simulink model "atm"  (R2017a)
settings: Solver=FixedStepDiscrete  StartTime=0.0  StopTime=15  FixedStep=0.1  RelTol=1e-3  EnableMultiTasking=on
settings Model: NumberOfSteps=10  Creator=thr  LastModifiedBy=thr
settings SolverCC: AutoInsertRateTranBlk=on
settings DataIOCC: LimitDataPoints=on
settings OptimizationCC: LifeSpan=inf
settings DebuggingCC: AllowSymbolicDim=off  SFUnexpectedBacktrackingDiag=warning  SFNoUnconditionalDefaultTransitionDiag=warning  SFExecutionAtInitializationDiag=none
settings GRTTargetCC: TargetLangStandard=C89/C90 (ANSI)  GeneratePreprocessorConditionals=Disable all
settings ConfigComp: CovMetricSettings=dw  CovHtmlReporting=on  CovSaveCumulativeToWorkspaceVar=on  CovSaveSingleToWorkspaceVar=on  CovShowResultsExplorer=off  CovExternalEMLEnable=off  CovSFcnEnable=off

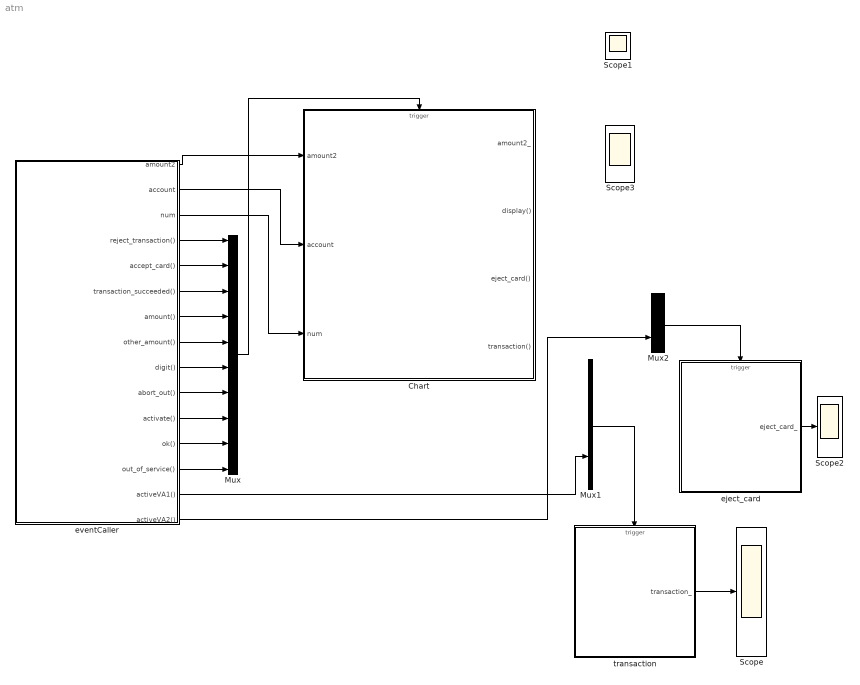
== system atm ==
  Chart : Stateflow chart  TreatAsAtomicUnit=on
  Mux : Mux  Inputs=10
  Mux1 : Mux  Inputs=2
  Mux2 : Mux  Inputs=2
  Scope : Scope
  Scope1 : Scope
  Scope2 : Scope
  Scope3 : Scope  NumInputPorts=2
  eject_card : Stateflow chart  TreatAsAtomicUnit=on
  eventCaller : Stateflow chart  TreatAsAtomicUnit=on
  transaction : Stateflow chart  TreatAsAtomicUnit=on
  wires:
  eventCaller/1(amount2) -> Chart/1(amount2)
  eventCaller/2(account) -> Chart/2(account)
  eventCaller/3(num) -> Chart/3(num)
  Mux/1 -> Chart/Trigger
  eventCaller/4(reject_transaction()) -> Mux/1
  eventCaller/5(accept_card()) -> Mux/2
  eventCaller/6(transaction_succeeded()) -> Mux/3
  eventCaller/7(amount()) -> Mux/4
  eventCaller/8(other_amount()) -> Mux/5
  eventCaller/9(digit()) -> Mux/6
  eventCaller/10(abort_out()) -> Mux/7
  eventCaller/11(activate()) -> Mux/8
  eventCaller/12(ok()) -> Mux/9
  eventCaller/13(out_of_service()) -> Mux/10
  Mux1/1 -> transaction/Trigger
  eventCaller/14(activeVA1()) -> Mux1/2
  transaction/1(transaction_) -> Scope/1
  eventCaller/15(activeVA2()) -> Mux2/2
  Mux2/1 -> eject_card/Trigger
  eject_card/1(eject_card_) -> Scope2/1

== stateflow chart atm/eventCaller ==
  state S1
  state S2
  state S3
  state S5
  state S4
  state S6
  state S10
  state S9
  state S8
  state S14
  state S7
  state S11
  (default) -> S1 : {activate, activeVA1,activeVA2}
  S2 -> S3 : after(1, sec)
      | {amount2=5000,
      | amount}
  S1 -> S2 : after(1, sec)
      | {accept_card,
      | account=2345}
  S3 -> S5 : after(1, sec)
      | {reject_transaction}
  S5 -> S4 : after(1, sec)
      | {num=5,
      | digit}
  S4 -> S6 : after(1, sec)
      | {num=0,
      | digit}
  S6 -> S7 : after(1, sec)
      | {num=0,
      | digit}
  S8 -> S9 : after(1, sec)
      | {num=5,
      | digit}
  S14 -> S8 : after(1, sec)
      | {reject_transaction}
  S7 -> S14 : after(1, sec)
      | {ok}
  S9 -> S10 : after(1, sec)
      | {ok}
  S10 -> S11 : after(1, sec)
      | {transaction_succeeded}
  data: amount2 output int32; account output int32; num output int32
  events: reject_transaction output FUNCTION_CALL_EVENT; accept_card output FUNCTION_CALL_EVENT; transaction_succeeded output FUNCTION_CALL_EVENT; amount output FUNCTION_CALL_EVENT; other_amount output FUNCTION_CALL_EVENT; digit output FUNCTION_CALL_EVENT; abort_out output FUNCTION_CALL_EVENT; activate output FUNCTION_CALL_EVENT; ok output FUNCTION_CALL_EVENT; out_of_service output FUNCTION_CALL_EVENT; activeVA1 output FUNCTION_CALL_EVENT; activeVA2 output FUNCTION_CALL_EVENT

== stateflow chart atm/transaction ==
  state A
    entry: transaction_=-1
  state B
    entry: transaction_=1
  (default) -> A : activeVA1
  A -> B : transaction
  B -> A : transaction
  data: transaction_ output int32
  events: transaction input FUNCTION_CALL_EVENT; activeVA1 input FUNCTION_CALL_EVENT

== stateflow chart atm/Chart ==
  state VERIFYING_CARD
    entry: fprintf('VERIFYING_CARD')
  state READ_AMOUNT
    entry: fprintf('READ_AMOUNT')
    state AMOUNT_SELECTION
      entry: fprintf('AMOUNT_SELECTION')
    state ENTER_AMOUNT
      entry: fprintf('ENTER_AMOUNT')
    (default) -> AMOUNT_SELECTION : {display_=1; display,
        | fprintf('<- display - Select amount')}
    AMOUNT_SELECTION -> ENTER_AMOUNT [order 2] : other_amount
        | {amount2_=0;
        | fprintf('other_amount ->')}
    ENTER_AMOUNT -> ENTER_AMOUNT [order 1] : digit{num_=num;
        | fprintf('digit - %d ->', num),
        | amount2_=amount2_*10+num_;}
  state VERIFYING_TRANSACTION
    entry: fprintf('VERIFYING_TRANSACTION')
  state CARD_RELEASED
    entry: fprintf('CARD_RELEASED')
  state OUT_OF_SERVICE
    entry: fprintf('OUT_OF_SERVICE')
  (default) -> VERIFYING_CARD : activate
  VERIFYING_CARD -> READ_AMOUNT : accept_card
      | {account_=account;
      | fprintf('accept_card ->')}
  AMOUNT_SELECTION -> VERIFYING_TRANSACTION [order 1] : amount
      | {transaction,
      | amount2_=amount2;
      | fprintf('amount - %d ->', amount2),
      | fprintf('<- transaction - %d', amount2_)}
  AMOUNT_SELECTION -> CARD_RELEASED [order 3] : abort_out
      | {fprintf('abort_out ->')}
  ENTER_AMOUNT -> VERIFYING_TRANSACTION [order 3] : ok{transaction,
      | fprintf('ok ->'),
      | fprintf('<- transaction - %d', amount2_)}
  ENTER_AMOUNT -> CARD_RELEASED [order 2] : abort_out
      | {fprintf('abort_out ->')}
  VERIFYING_TRANSACTION -> ENTER_AMOUNT [order 1] : reject_transaction
      | {display_=-1; display,
      | amount2_=0;
      | fprintf('reject_transaction ->')
      | fprintf('<- display - Limit exceeded')}
  READ_AMOUNT -> OUT_OF_SERVICE : out_of_service
      | {fprintf('out_of_service ->')}
  VERIFYING_TRANSACTION -> CARD_RELEASED [order 2] : transaction_succeeded
      | {eject_card
      | fprintf('transaction_succeeded ->')
      | fprintf('<- eject_card')}
  data: amount2 input int32; account input int32; num input int32; account_ local int32; amount2_ output int32; num_ local int32; display_ local int32
  events: reject_transaction input FUNCTION_CALL_EVENT; accept_card input FUNCTION_CALL_EVENT; display output FUNCTION_CALL_EVENT; transaction_succeeded input FUNCTION_CALL_EVENT; eject_card output FUNCTION_CALL_EVENT; amount input FUNCTION_CALL_EVENT; other_amount input FUNCTION_CALL_EVENT; digit input FUNCTION_CALL_EVENT; abort_out input FUNCTION_CALL_EVENT; transaction output FUNCTION_CALL_EVENT; activate input FUNCTION_CALL_EVENT; ok input FUNCTION_CALL_EVENT; out_of_service input FUNCTION_CALL_EVENT

== stateflow chart atm/eject_card ==
  state A
    entry: eject_card_=-1
  state B
    entry: eject_card_=1
  (default) -> A : activeVA2
  A -> B : eject_card
  B -> A : eject_card
  data: eject_card_ output int32
  events: eject_card input FUNCTION_CALL_EVENT; activeVA2 input FUNCTION_CALL_EVENT
